simulink model "mBlocksAndObserver"  (R2024a)
settings: Solver=VariableStepAuto  StartTime=0.0  StopTime=10.0  RelTol=1e-3
undefined symbols (not defined in the file): physconst
libraries: radarlib x1, matrix_library x1
settings Model: Creator=neham  LastModifiedBy=neham

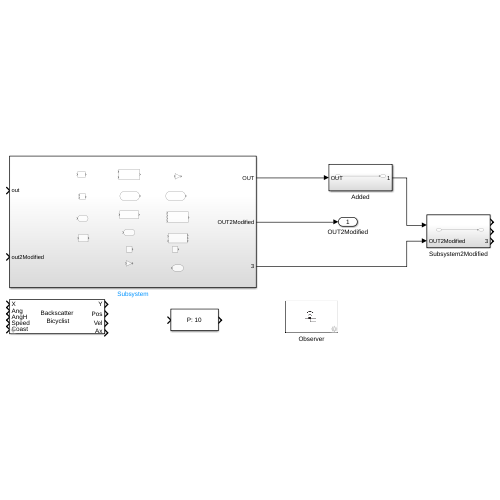
[thumbnail: Simulink's stored preview of the top-level diagram]
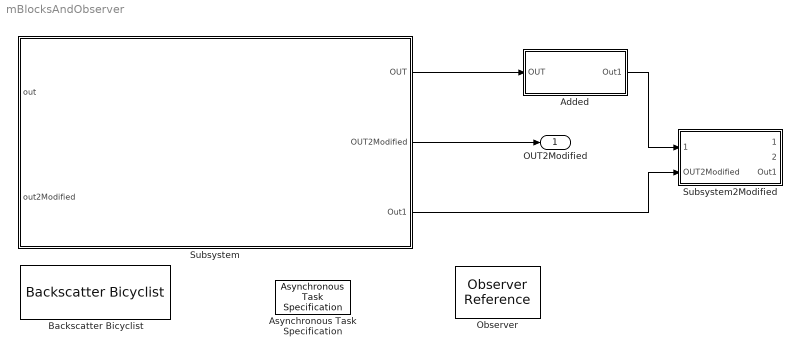
== system mBlocksAndObserver ==
  Added : Subsystem
  Asynchronous Task Specification : AsynchronousTaskSpecification
  Backscatter Bicyclist : radarlib/Backscatter Bicyclist  NumWheelSpokes=20  GearTransmissionRatio=1.5  OperatingFrequency=77e9  InitialPosition=[0;0;0]  InitialHeading=0  InitialSpeed=4  PropagationSpeed=physconst('lightspeed')  RCSPatternSource=Auto  AzimuthAngles=-180:180  ElevationAngles=0  RCSPattern=backscatterBicyclist.defaultRCSPattern  SimulateUsing=Interpreted execution
  Observer : ObserverReference
  Subsystem : Subsystem
  Subsystem2Modified : Subsystem
  OUT2Modified : Outport
  wires:
  Subsystem/1(OUT) -> Added/1(OUT)
  Added/1(Out1) -> Subsystem2Modified/1
  Subsystem/2(OUT2Modified) -> OUT2Modified/1
  Subsystem/3(Out1) -> Subsystem2Modified/2(OUT2Modified)

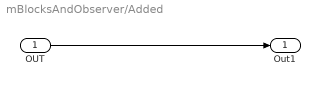
== system mBlocksAndObserver/Added ==
  OUT : Inport
  Out1 : Outport
  wires:
  OUT/1 -> Out1/1

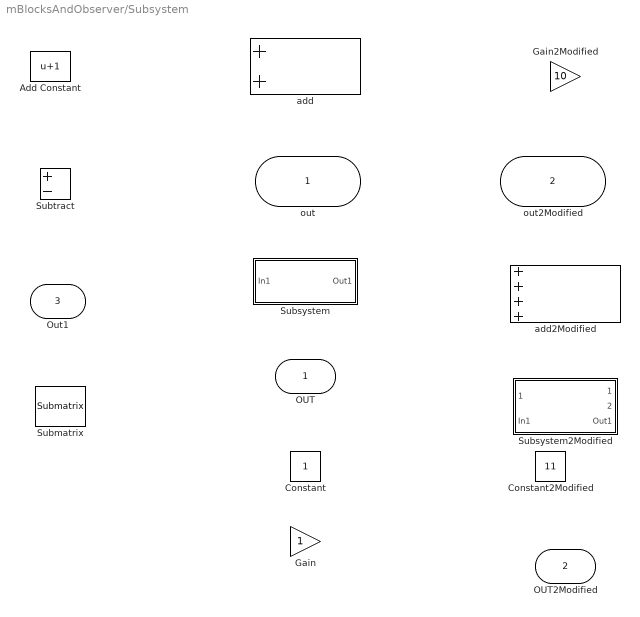
== system mBlocksAndObserver/Subsystem ==
  out : Inport
  out2Modified : Inport  Port=2
  Add Constant : Bias  Bias=1  SaturateOnIntegerOverflow=off
  Constant : Constant
  Constant2Modified : Constant  Value=11
  Gain : Gain
  Gain2Modified : Gain  Gain=10
  Submatrix : matrix_library/Submatrix  RowSpan=Range of rows  RowStartMode=First  RowStartIndex=1  RowEndMode=Last  RowEndIndex=1  ColSpan=Range of columns  ColStartMode=First  ColStartIndex=1  ColEndMode=Last  ColEndIndex=1
  Subsystem : Subsystem
  Subsystem2Modified : Subsystem
  Subtract : Sum  Inputs=+-
  add : Sum
  add2Modified : Sum  Inputs=++++
  OUT : Outport
  OUT2Modified : Outport  Port=2
  Out1 : Outport  Port=3  VectorParamsAs1DForOutWhenUnconnected=off

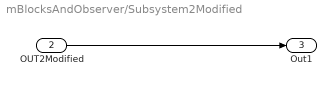
== system mBlocksAndObserver/Subsystem2Modified ==
  OUT2Modified : Inport  Port=2
  Out1 : Outport  Port=3
  wires:
  OUT2Modified/1 -> Out1/1

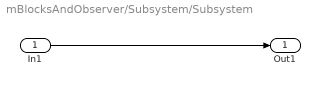
== system mBlocksAndObserver/Subsystem/Subsystem ==
  In1 : Inport
  Out1 : Outport
  wires:
  In1/1 -> Out1/1

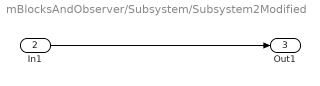
== system mBlocksAndObserver/Subsystem/Subsystem2Modified ==
  In1 : Inport  Port=2
  Out1 : Outport  Port=3
  wires:
  In1/1 -> Out1/1
